simulink model "PC_CONTROL_STATION"  (R2023b)
settings: Solver=FixedStepAuto  StartTime=0.0  StopTime=inf  RelTol=1e-3  EnableMultiTasking=on
InitFcn:
  | if RUN_MODE~=5
  |     % clear rpi;
  |     rpi = raspberrypi(CAR_IP, 'pi', 'LabControl');
  |     stopModel(rpi,'CAR_CONTROL_SYSTEM')
  |     while isModelRunning(rpi,'CAR_CONTROL_SYSTEM')
  |          stopModel(rpi,'CAR_CONTROL_SYSTEM')
  |     end
  |     runModel(rpi,'CAR_CONTROL_SYSTEM')
  |      while isModelRunning(rpi,'CAR_CONTROL_SYSTEM')==false
  |          runModel(rpi,'CAR_CONTROL_SYSTEM')
  |      end
  |      % clear rpi;
  | end
StopFcn:
  | if RUN_MODE~=5
  |    clear rpi;
  |    rpi = raspberrypi(CAR_IP, 'pi', 'LabControl');
  |    stopModel(rpi,'CAR_CONTROL_SYSTEM')
  |    while isModelRunning(rpi,'CAR_CONTROL_SYSTEM')
  |    end
  |    clear rpi;
  | end
model workspace (MAT data in the model file):
  SL_ROS_VariableLengthArrays_MaxSizes : object (value not decoded)
values from neighbouring files (symbols this model uses):
  data = theClient.GetLastFrameOfData()    [FuncMotive.m]
undefined symbols (not defined in the file or in its folder): CONTROL, CONTROL_INI, data_SL_Info, MD25, MSG, SAMPLING_TIME, Standard_Devices, SYSID_INPUT, TCP_Protocol, UDP_Protocol
libraries: simulink x51, sldrtlib x46, dspsigattribs x7, ros2lib x3, ctrlSharedLib x2, aerolibanimutils x1
(part 8 of 8)

== matlab function PC_CONTROL_STATION/STATE MACHINE/STATE MACHINE UPDATE ==
  data: CONTROL_IN input Bus: CONTROL_Bus; CONTROL output Bus: CONTROL_Bus; MSG_IN input; MSG output Bus: MSG_Bus; DATA_DIFF output
function [CONTROL,MSG,DATA_DIFF] = STATE_MACHINE(CONTROL_IN,MSG_IN)

%--------------------------------------------------------------
% COPY BUSES
%--------------------------------------------------------------
CONTROL = CONTROL_IN;
MSG = MSG_IN;
DATA_DIFF = 0;
% NUM_MSG_RX = 0;
% NUM_MSG_TX = 0;

%--------------------------------------------------------------
% TIMING
%--------------------------------------------------------------
% SAMPLING TIME
SAMPLING_TIME = CONTROL.PARAM.COMM_SAMPLING_TIME; % s
% 6-bit SAMPLING COUNTER
SAMPLING_COUNT = CONTROL.STATE.SAMPLING_COUNT;
SAMPLING_COUNT = SAMPLING_COUNT + uint8(1);
if SAMPLING_COUNT > uint8(63) 
    SAMPLING_COUNT = uint8(0);
end
CONTROL.STATE.SAMPLING_COUNT = SAMPLING_COUNT;
% TIMER
TIMER = CONTROL.STATE.TIMER;

%--------------------------------------------------------------
% SYSTEM OPERATION STATUS
%--------------------------------------------------------------
% / 0. BOOTING   / 1. SENSOR CALIBRATION / 2. READY /
% / 3. OPEN LOOP / 4. FORWARD VELOCITY AND YAW ANGLE / 
% / 5. FORWARD VELOCITY AND YAW RATE / 6. NAVIGATION / 
% / 7. WALL FOLLOWER / 8. WALL-FOLLOWER COMPETITION / 
% / 9. NAVIGATION COMPETITION / 10. STOP
CURRENT_STATUS_SYS = CONTROL.STATE.CURRENT_STATUS_SYS;

%--------------------------------------------------------------
% PC OPERATION STATUS
%--------------------------------------------------------------
% / 0. CONTROL CONFIGURATION   / 1. WAITING FOR RPI SET UP  /
% / 2. MONITORIZATION / 3. STOP /
CURRENT_STATUS_PC = CONTROL.STATE.CURRENT_STATUS_PC;
NEXT_STATUS = CURRENT_STATUS_PC;

%--------------------------------------------------------------
% UART MODE
%--------------------------------------------------------------
%--------------------------------------------------------------
% COMMUNICATIONS
%--------------------------------------------------------------
% / 0. NOT ENABLED / 1. ENABLED
UART_MODE = CONTROL.STATE.UART_MODE;

%--------------------------------------------------------------
% PERSISTENT VARIABLES
%--------------------------------------------------------------
persistent PC_MSG_BUFFER COMM_FAILED nn initialize
if isempty(initialize)
    PC_MSG_BUFFER = uint8(1);
    COMM_FAILED = uint8(0);
    nn = 0;
    initialize = 1;
end

%--------------------------------------------------------------
% STATUS UPDATE
%--------------------------------------------------------------
switch CURRENT_STATUS_PC
    
    %----------------------------------------------------------------------
    case 0 % CONTROL CONFIGURATION
    %----------------------------------------------------------------------
        BUFFER_RX = MSG.RX_BUFFER;
        NUM_MSG_RX = double(BUFFER_RX(1));
        if NUM_MSG_RX > 0
            HEADER_RX = BUFFER_RX(1:2*NUM_MSG_RX+1);
            MSG_LEN_RX = double(HEADER_RX(3:2:end));
            DATA_LEN_RX = sum(MSG_LEN_RX);
            % DATA_RX = BUFFER_RX(2*NUM_MSG_RX+2:2*NUM_MSG_RX+2+DATA_LEN_RX-1);
            % DATA_RX = DATA_RX(MSG_LEN_RX(1)+1:end);
            DATA_RX = BUFFER_RX(2*NUM_MSG_RX+MSG_LEN_RX(1)+2:2*NUM_MSG_RX+2+DATA_LEN_RX-1);
            DATA_LEN_RX = length(DATA_RX);
        else
            DATA_LEN_RX = 0;
            DATA_RX = uint8(0);
        end
        BUFFER_TX = MSG.TX_BUFFER;
        NUM_MSG_TX = double(BUFFER_TX(1));
        if NUM_MSG_TX > 0
            HEADER_TX = BUFFER_TX(1:2*NUM_MSG_TX+1);
            MSG_LEN_TX = double(HEADER_TX(3:2:end));
            DATA_LEN_TX = sum(MSG_LEN_TX);
            % DATA_TX = BUFFER_TX(2*NUM_MSG_TX+2:2*NUM_MSG_TX+2+DATA_LEN_TX-1);
            % DATA_TX = DATA_TX(MSG_LEN_TX(1)+1:end);
            DATA_TX = BUFFER_TX(2*NUM_MSG_TX+MSG_LEN_TX(1)+2:2*NUM_MSG_TX+2+DATA_LEN_TX-1);
            DATA_LEN_TX = length(DATA_TX);
        else
            DATA_LEN_TX = 0;
            DATA_TX = uint8(0);
        end
        % Same message check
        if DATA_LEN_TX*DATA_LEN_RX > 0 && DATA_LEN_TX == DATA_LEN_RX
            DATA_DIFF = sum(abs(double(DATA_TX-DATA_RX)));
        % Different messages yet
        % elseif DATA_LEN_TX*DATA_LEN_RX > 0
        %         % DATA_LEN_RX
        %         % DATA_LEN_TX
        %     DATA_DIFF = 1;
        %At least one message not received
        else
            DATA_DIFF = 1;
            % end
        end

        if PC_MSG_BUFFER <= size(MSG.MSG_ID_LIST,2)
            MSG.TX_ID = MSG.MSG_ID_LIST(:,PC_MSG_BUFFER);
            if DATA_DIFF==0
                [BUFFER_TX(4) BUFFER_RX(4)]
                PC_MSG_BUFFER = PC_MSG_BUFFER + 1;
                MSG.TX_BUFFER = zeros(1400,1,'uint8');
                COMM_FAILED = uint8(0);
                nn = 0;
            elseif (nn >= 400) && DATA_DIFF>0
                NEXT_STATUS = uint8(3); % STOP
                COMM_FAILED = uint8(1);
                nn = 0;
            else
                nn = nn + 1;
            end

        else
            NEXT_STATUS = uint8(1); % WAITING FOR RPI SET UP
            PC_MSG_BUFFER = uint8(1);
            nn = 0;
            COMM_FAILED = uint8(0);
        end
        
        
        
    %----------------------------------------------------------------------
    case 1 % WAITING FOR RPI SET UP
    %----------------------------------------------------------------------
        if (UART_MODE==0)
            MSG.TX_ID = uint8([2 0 0 0 0 0 0 0]');
        end
        if ((CURRENT_STATUS_SYS >= 3) && (CURRENT_STATUS_SYS ~= 11))
            NEXT_STATUS = uint8(2); % MONITORIZATION
        end

    %----------------------------------------------------------------------
    case 2 % MONITORIZATION
    %----------------------------------------------------------------------
        if (UART_MODE==0)
            MSG.TX_ID = uint8([2 0 0 0 0 0 0 0]');
        end
        if (CURRENT_STATUS_SYS == 0)
            NEXT_STATUS = uint8(3); % STOP
        end
    %----------------------------------------------------------------------
    case 3 % STOP
    %----------------------------------------------------------------------
        MSG.TX_ID = uint8([0 0 0 0 0 0 0 0]');
        TIMER = TIMER + SAMPLING_TIME;
        if TIMER > 5
            TIMER = 0;
            NEXT_STATUS = uint8(0);
        end
        nn = 0;
end

%--------------------------------------------------------------
% CONTROL BUS UPDATE
%--------------------------------------------------------------
CONTROL.STATE.CURRENT_STATUS_PC = NEXT_STATUS;
CONTROL.STATE.TIMER = TIMER;
CONTROL.STATE.COMM_STATUS = COMM_FAILED;

== matlab function PC_CONTROL_STATION/PC TARGETS/PC TARGETS/YAW ANGLE TARGET/ PULSE GENERATION ==
  data: CONTROL input Bus: CONTROL_Bus; YAW_ANG_REF output
function YAW_ANG_REF = PULSE_GEN(CONTROL)
    
persistent TIMER initialize
if isempty(initialize)
    TIMER = 0;
    initialize = 1;
end

% SAMPLING TIME
SAMPLING_TIME = CONTROL.PARAM.SAMPLING_TIME; % s

%% OPERATION MODE
% / 0. BOOTING   / 1. SENSOR CALIBRATION / 2. READY
% / 3. OPEN LOOP / 4. ATTITUDE / 5. VELOCITY / 6. NAVIGATION / 
% / 7. WALL FOLLOWER / 8. WALL-FOLLOWER COMPETITION / 
% / 9. NAVIGATION COMPETITION / 10. STOP
CURRENT_STATUS = CONTROL.STATE.CURRENT_STATUS_SYS;
PREVIOUS_STATUS = CONTROL.STATE.PREVIOUS_STATUS;

if (CURRENT_STATUS == 4) && (PREVIOUS_STATUS == 4)   
    if TIMER > 3
        YAW_ANG_REF = 0;
    elseif TIMER < 0.5
        YAW_ANG_REF = 0;
        TIMER = TIMER + SAMPLING_TIME;
    else % 0.5 <= TIMER <= 3
        YAW_ANG_REF = 60*pi/180;
        TIMER = TIMER + SAMPLING_TIME;
    end
else
    YAW_ANG_REF = 0;
    TIMER = 0;
end

== matlab function PC_CONTROL_STATION/MONITORING/SYSTEM IDENTIFICATION/Second-order equation1 ==
  data: b input; r1 output; c input; r2 output
function [r1,r2] = sol_2ord_eq(b,c)
r1 = (-b+sqrt(abs(b^2-4*c)))/2;
r2 = (-b-sqrt(abs(b^2-4*c)))/2;
return

== matlab function PC_CONTROL_STATION/PC TARGETS/PC TARGETS/OPL TARGETS/VOLTAGE PULSE GENERATION ==
  data: CONTROL input Bus: CONTROL_Bus; MOTOR_VOLT_TARGET output
function MOTOR_VOLT_TARGET = PULSE_VOLT_GEN(CONTROL)
    
persistent TIMER initialize
if isempty(initialize)
    TIMER = 0;
    initialize = 1;
end

% SAMPLING TIME
SAMPLING_TIME = CONTROL.PARAM.SAMPLING_TIME; % s

%% OPERATION MODE
% / 0. BOOTING   / 1. SENSOR CALIBRATION / 2. READY
% / 3. OPEN LOOP / 4. ATTITUDE / 5. VELOCITY / 6. NAVIGATION / 
% / 7. WALL FOLLOWER / 8. WALL-FOLLOWER COMPETITION / 
% / 9. NAVIGATION COMPETITION / 10. STOP
CURRENT_STATUS = CONTROL.STATE.CURRENT_STATUS_SYS;
PREVIOUS_STATUS = CONTROL.STATE.PREVIOUS_STATUS;

if (CURRENT_STATUS == 3)&&(PREVIOUS_STATUS == 3)   
    if TIMER > 6
        MOTOR_VOLT_TARGET = 0;
    elseif TIMER < 5
        MOTOR_VOLT_TARGET = 0;
        TIMER = TIMER + SAMPLING_TIME;
    else % 5 <= TIMER <= 6
        MOTOR_VOLT_TARGET = 4;
        TIMER = TIMER + SAMPLING_TIME;
    end
else
    MOTOR_VOLT_TARGET = 0;
    TIMER = 0;
end
